simulink library "walkingRobotUtils"  (R2019a)
settings: Solver=VariableStepAuto  StartTime=0.0  StopTime=10.0  RelTol=1e-3
undefined symbols (not defined in the file): ankle_servo_kd, ankle_servo_ki, ankle_servo_kp, deriv_filter_coeff, joint_damping, joint_stiffness, lower_leg_length, max_torque, motion_time_constant, motor_constant, motor_inertia, upper_leg_length
libraries: nesl_utility x17, fl_lib x7, $bdroot x5, sm_lib x4, ee_lib x3, simulink x2, simulink_extras x2, robotcorelib x1, Multibody_Multiphysics_Lib x1
settings Model: Creator=scastro  LastModifiedBy=michaelmcgeehan
settings DataIOCC: ReturnWorkspaceOutputs=off
settings DebuggingCC: ArithmeticOperatorsInVariantConditions=warning
settings SFSimCC: SimUseLocalCustomCode=off
settings RTWCC: RTWUseLocalCustomCode=off
settings CodeAppCC: StateflowObjectComments=on

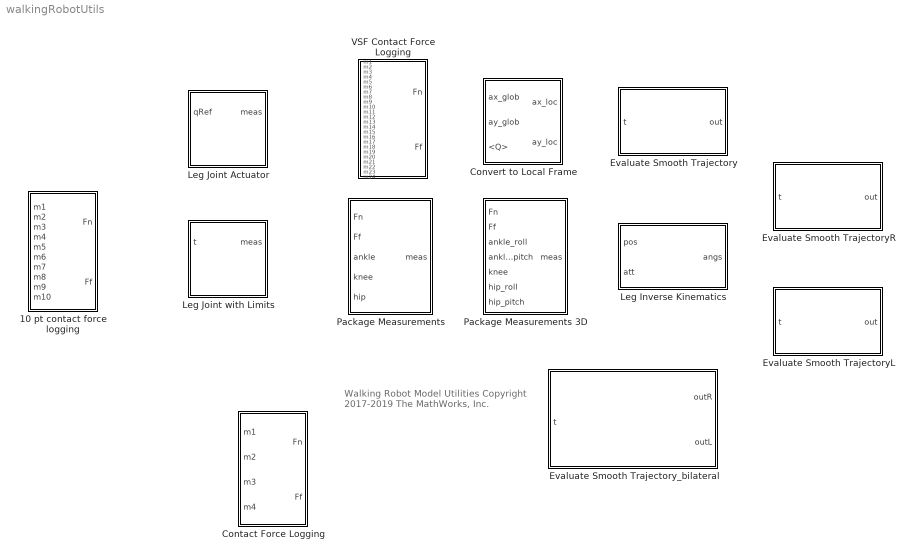
== system walkingRobotUtils ==
  note: Walking Robot Model Utilities
      |
      | Copyright 2017-2019 The MathWorks, Inc.
  10 pt contact force logging : Subsystem  AncestorBlock=walkingRobotUtils/VSF Contact Force Logging
  Contact Force Logging : Subsystem  AncestorBlock=walkingRobotUtils/VSF Contact Force Logging
  Convert to Local Frame : Subsystem
  Evaluate Smooth Trajectory : MATLAB Function  TreatAsAtomicUnit=on
  Evaluate Smooth TrajectoryL : MATLAB Function  TreatAsAtomicUnit=on
  Evaluate Smooth TrajectoryR : MATLAB Function  TreatAsAtomicUnit=on
  Evaluate Smooth Trajectory_bilateral : MATLAB Function  TreatAsAtomicUnit=on
  Leg Inverse Kinematics : MATLAB Function  TreatAsAtomicUnit=on
  Leg Joint Actuator : Subsystem  Variant=on  mask(Leg Joint Actuator){k=joint_stiffness, d=joint_damping, initAngle=0, Tf=motion_time_constant, Kp=ankle_servo_kp, Ki=ankle_servo_ki, Kd=ankle_servo_kd, N=deriv_filter_coeff, Tmax=max_torque}
      mask prompts: k "Joint Stiffness [N*m/rad]"; d "Joint Damping [N*m/(rad/s)]"; initAngle "Initial Joint Angle"; Tf "Motion Time Constant"; Kp "Servo Proportional Gain"; Ki "Servo Integral Gain"; Kd "Servo Derivative Gain"; N "Servo Filter Coefficient"; Tmax "Maximum Torque"
      mask DialogControl Container7 Prompt: Mechanics
      mask DialogControl Container4 Prompt: Controller
  Leg Joint with Limits : Subsystem  VariantControl=actuatorType == 2  mask(Leg Joint with Limits){k=1, d=0, initAngle=0, eqAngle=0, upperLimit=0, lowerLimit=-pi/8, jointLimitStiffness=100, jointLimitDamping=10}
      mask prompts: k "Joint Stiffness [N*m/rad]"; d "Joint Damping [N*m/(rad/s)]"; initAngle "Initial Angle [rad]"; eqAngle "Equilibrium Angle [rad]"; upperLimit "Upper Angle Limit [rad]"; lowerLimit "Lower Angle Limit [rad]"; jointLimitStiffness "Joint Limit Stiffness [N*m/rad]"; jointLimitDamping "Joint Limit Damping [N*m/(rad/s)]"
      mask help: Torque-actuated revolute joint with limits and instrumented measurements.
      mask DialogControl DynamicsTab Prompt: Dynamics
      mask DialogControl LimitsTab Prompt: Limits
  Package Measurements 3D : Subsystem
  Package Measurements : Subsystem
  VSF Contact Force Logging : Subsystem

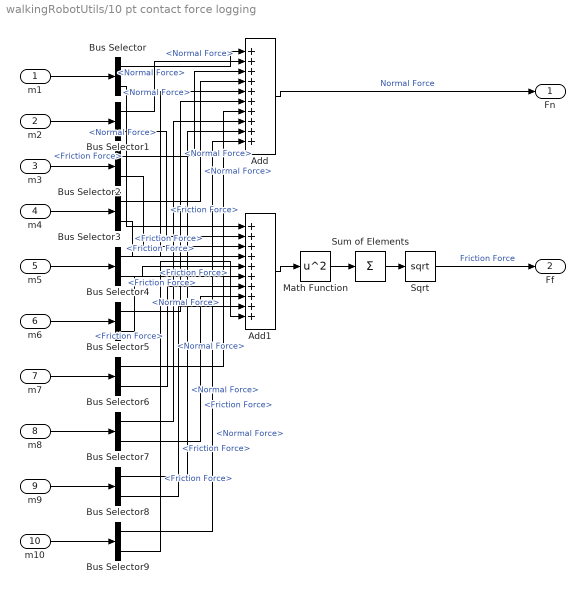
== system walkingRobotUtils/10 pt contact force logging ==
  m1 : Inport
  m2 : Inport  Port=2
  m3 : Inport  Port=3
  m4 : Inport  Port=4
  m5 : Inport  Port=5
  m6 : Inport  Port=6
  m7 : Inport  Port=7
  m8 : Inport  Port=8
  m9 : Inport  Port=9
  m10 : Inport  Port=10
  Add : Sum  Inputs=10
  Add1 : Sum  Inputs=10
  Bus Selector{,1..9} (10 alike) : BusSelector  OutputSignals=Normal Force,Friction Force
  Math Function : Math  Operator=square  SaturateOnIntegerOverflow=on
  Sqrt : Sqrt  SaturateOnIntegerOverflow=on
  Sum of Elements : Sum  Inputs=+
  Fn : Outport
  Ff : Outport  Port=2
  wires:
  m1/1 -> Bus Selector/1
  m2/1 -> Bus Selector1/1
  m3/1 -> Bus Selector2/1
  m4/1 -> Bus Selector3/1
  Bus Selector/1 -> Add/1  "<Normal Force>"
  Bus Selector1/1 -> Add/2  "<Normal Force>"
  Bus Selector2/1 -> Add/3  "<Normal Force>"
  Bus Selector3/1 -> Add/4  "<Normal Force>"
  Bus Selector/2 -> Add1/1  "<Friction Force>"
  Bus Selector1/2 -> Add1/2  "<Friction Force>"
  Bus Selector2/2 -> Add1/3  "<Friction Force>"
  Bus Selector3/2 -> Add1/4  "<Friction Force>"
  Add/1 -> Fn/1  "Normal Force"
  Add1/1 -> Math Function/1
  Math Function/1 -> Sum of Elements/1
  Sum of Elements/1 -> Sqrt/1
  Sqrt/1 -> Ff/1  "Friction Force"
  m5/1 -> Bus Selector4/1
  m6/1 -> Bus Selector5/1
  m7/1 -> Bus Selector6/1
  m8/1 -> Bus Selector7/1
  m9/1 -> Bus Selector8/1
  m10/1 -> Bus Selector9/1
  Bus Selector4/1 -> Add/5  "<Normal Force>"
  Bus Selector5/1 -> Add/6  "<Normal Force>"
  Bus Selector6/1 -> Add/7  "<Normal Force>"
  Bus Selector7/1 -> Add/8  "<Normal Force>"
  Bus Selector8/1 -> Add/9  "<Normal Force>"
  Bus Selector9/1 -> Add/10  "<Normal Force>"
  Bus Selector4/2 -> Add1/5  "<Friction Force>"
  Bus Selector5/2 -> Add1/6  "<Friction Force>"
  Bus Selector6/2 -> Add1/7  "<Friction Force>"
  Bus Selector7/2 -> Add1/8  "<Friction Force>"
  Bus Selector8/2 -> Add1/9  "<Friction Force>"
  Bus Selector9/2 -> Add1/10  "<Friction Force>"

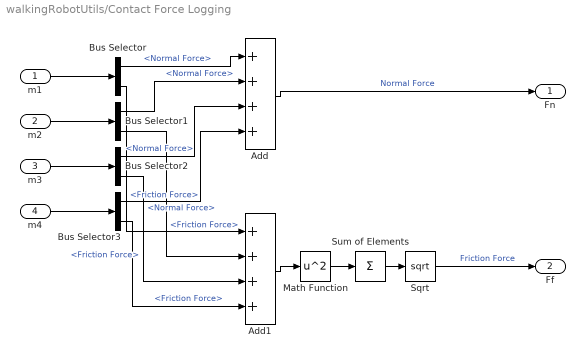
== system walkingRobotUtils/Contact Force Logging ==
  m1 : Inport
  m2 : Inport  Port=2
  m3 : Inport  Port=3
  m4 : Inport  Port=4
  Add : Sum  Inputs=4
  Add1 : Sum  Inputs=4
  Bus Selector{,1..3} (4 alike) : BusSelector  OutputSignals=Normal Force,Friction Force
  Math Function : Math  Operator=square  SaturateOnIntegerOverflow=on
  Sqrt : Sqrt  SaturateOnIntegerOverflow=on
  Sum of Elements : Sum  Inputs=+
  Fn : Outport
  Ff : Outport  Port=2
  wires:
  m1/1 -> Bus Selector/1
  m2/1 -> Bus Selector1/1
  m3/1 -> Bus Selector2/1
  m4/1 -> Bus Selector3/1
  Bus Selector/1 -> Add/1  "<Normal Force>"
  Bus Selector1/1 -> Add/2  "<Normal Force>"
  Bus Selector2/1 -> Add/3  "<Normal Force>"
  Bus Selector3/1 -> Add/4  "<Normal Force>"
  Bus Selector/2 -> Add1/1  "<Friction Force>"
  Bus Selector1/2 -> Add1/2  "<Friction Force>"
  Bus Selector2/2 -> Add1/3  "<Friction Force>"
  Bus Selector3/2 -> Add1/4  "<Friction Force>"
  Add/1 -> Fn/1  "Normal Force"
  Add1/1 -> Math Function/1
  Math Function/1 -> Sum of Elements/1
  Sum of Elements/1 -> Sqrt/1
  Sqrt/1 -> Ff/1  "Friction Force"

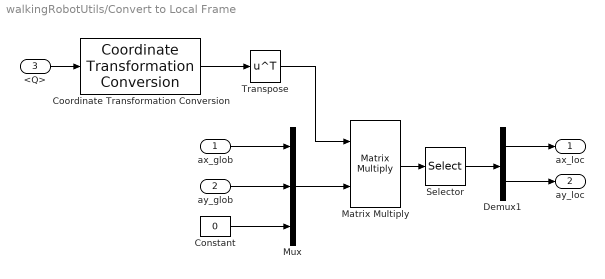
== system walkingRobotUtils/Convert to Local Frame ==
  ax_glob : Inport
  ay_glob : Inport  Port=2
  <Q> : Inport  Port=3
  Constant : Constant  Value=0
  Coordinate Transformation Conversion : robotcorelib/Coordinate Transformation Conversion  InputRepresentation=Quaternion  InputEulerSequence=ZYX  ShowTrVecInputPort=on  OutputRepresentation=Rotation Matrix  OutputEulerSequence=ZYX  ShowTrVecOutputPort=on  SimulateUsing=Interpreted execution
      settings: SourceProductBaseCode=RO
  Demux1 : Demux  Outputs=2
  Matrix Multiply : Product  Multiplication=Matrix(*)
  Mux : Mux  Inputs=3
  Selector : Selector  InputPortWidth=3  IndexOptions=Index vector (dialog)  Indices=[1 2]  OutputSizes=1
  Transpose : Math  Operator=transpose  SaturateOnIntegerOverflow=on
  ax_loc : Outport
  ay_loc : Outport  Port=2
  wires:
  Mux/1 -> Matrix Multiply/2
  Demux1/2 -> ay_loc/1
  ay_glob/1 -> Mux/2
  <Q>/1 -> Coordinate Transformation Conversion/1
  Selector/1 -> Demux1/1
  Matrix Multiply/1 -> Selector/1
  Constant/1 -> Mux/3
  ax_glob/1 -> Mux/1
  Demux1/1 -> ax_loc/1
  Coordinate Transformation Conversion/1 -> Transpose/1
  Transpose/1 -> Matrix Multiply/1

== system walkingRobotUtils/Leg Joint Actuator ==
  note: 1) Add Subsystem or Model blocks as valid variant choices.
      | 2) You cannot connect blocks at this level. At simulation, connectivity is automatically
      | determined, based on the active variant and port name matching.
  qRef : Inport
  Motion : Subsystem  VariantControl=actuatorType == 1
  Motor : Subsystem  VariantControl=actuatorType == 3
  Torque : Subsystem  VariantControl=actuatorType == 2
  B : PMIOPort  Side=Left
  F : PMIOPort  Port=2  Side=Right
  meas : Outport

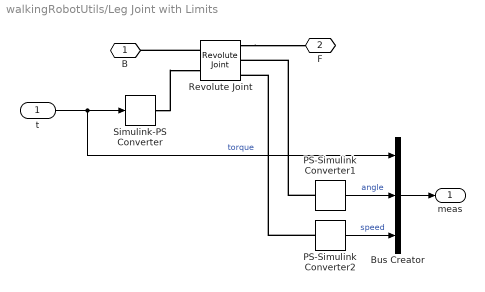
== system walkingRobotUtils/Leg Joint with Limits ==
  t : Inport
  Bus Creator : BusCreator  Inputs=3
  PS-Simulink Converter1 : nesl_utility/PS-Simulink Converter  PhysicalDomain=network_engine_domain  SubClassName=ps_output  LeftPortType=input  RightPortType=output  PseudoPeriodic=off  Frequencies=[]  Unit=rad  AffineConversion=off
  PS-Simulink Converter2 : nesl_utility/PS-Simulink Converter  PhysicalDomain=network_engine_domain  SubClassName=ps_output  LeftPortType=input  RightPortType=output  PseudoPeriodic=off  Frequencies=[]  Unit=rad/s  AffineConversion=off
  Revolute Joint : sm_lib/Joints/Revolute Joint  SenseConstraintForce=off  SenseConstraintForceX=off  SenseConstraintForceY=off  SenseConstraintForceZ=off  SenseConstraintTorque=off  SenseConstraintTorqueX=off  SenseConstraintTorqueY=off  SenseConstraintTorqueZ=off  SenseTotalForce=off  SenseTotalForceX=off  SenseTotalForceY=off  SenseTotalForceZ=off  SenseTotalTorque=off  SenseTotalTorqueX=off  SenseTotalTorqueY=off  SenseTotalTorqueZ=off  CompositeWrenchDir=FollowerOnBase  CompositeWrenchFrame=BaseFrame  EquilibriumPosition=eqAngle  EquilibriumPositionUnits=rad  SpringStiffness=k  SpringStiffnessUnits=N*m/rad  DampingCoefficient=d  DampingCoefficientUnits=N*m/(rad/s)  TorqueActuationMode=InputTorque  MotionActuationMode=ComputedMotion  SensePosition=on  SenseVelocity=on  SenseAcceleration=off  SenseTorqueForce=off  SenseLowerLimitTorqueForce=off  SenseUpperLimitTorqueForce=off  LowerLimitSpecify=on  LowerLimitBound=lowerLimit  LowerLimitBoundUnits=rad  LowerLimitStiffness=jointLimitStiffness  LowerLimitStiffnessUnits=N*m/rad  LowerLimitDamping=jointLimitDamping  LowerLimitDampingUnits=N*m/(rad/s)  LowerLimitTransitionRegionWidth=1  LowerLimitTransitionRegionWidthUnits=deg  UpperLimitSpecify=on  UpperLimitBound=upperLimit  UpperLimitBoundUnits=rad  UpperLimitStiffness=jointLimitStiffness  UpperLimitStiffnessUnits=N*m/rad  UpperLimitDamping=jointLimitDamping  UpperLimitDampingUnits=N*m/(rad/s)  UpperLimitTransitionRegionWidth=1  UpperLimitTransitionRegionWidthUnits=deg  PositionTargetSpecify=on  PositionTargetPriority=High  PositionTargetValue=initAngle  PositionTargetValueUnits=rad  VelocityTargetSpecify=off  VelocityTargetPriority=High  VelocityTargetValue=0  VelocityTargetValueUnits=deg/s
  Simulink-PS Converter : nesl_utility/Simulink-PS Converter  PhysicalDomain=network_engine_domain  SubClassName=ps_input  LeftPortType=input  RightPortType=output  PseudoPeriodic=off  Frequencies=[]  NoiseDistribution=none  NoiseParameters=[]  Unit=N*m  AffineConversion=off  FilteringAndDerivatives=provide  SimscapeFilterOrder=2  InputFilterTimeConstant=motion_time_constant  UdotUserProvided=0
  B : PMIOPort  Side=Left
  F : PMIOPort  Port=2  Side=Right
  meas : Outport
  wires:
  PS-Simulink Converter2/1 -> Bus Creator/3  "speed"
  t/1 -> Simulink-PS Converter/1, Bus Creator/1  "torque"
  Bus Creator/1 -> meas/1
  PS-Simulink Converter1/1 -> Bus Creator/2  "angle"
  connections:
  PS-Simulink Converter2/LConn1 -- Revolute Joint/RConn3
  Simulink-PS Converter/RConn1 -- Revolute Joint/LConn2
  Revolute Joint/RConn1 -- F/RConn1
  Revolute Joint/LConn1 -- B/RConn1
  PS-Simulink Converter1/LConn1 -- Revolute Joint/RConn2

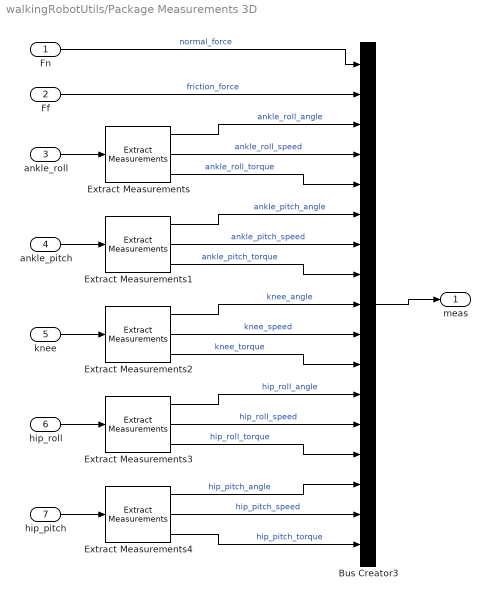
== system walkingRobotUtils/Package Measurements 3D ==
  Fn : Inport
  Ff : Inport  Port=2
  ankle_roll : Inport  Port=3
  ankle_pitch : Inport  Port=4
  knee : Inport  Port=5
  hip_roll : Inport  Port=6
  hip_pitch : Inport  Port=7
  Bus Creator3 : BusCreator  Inputs=17
  Extract Measurements{,1..4} (5 alike) : $bdroot/Package  Measurements/Extract Measurements  SystemSampleTime=-1
  meas : Outport
  wires:
  Extract Measurements4/2 -> Bus Creator3/16  "hip_pitch_speed"
  Extract Measurements3/2 -> Bus Creator3/13  "hip_roll_speed"
  Extract Measurements2/2 -> Bus Creator3/10  "knee_speed"
  Extract Measurements2/1 -> Bus Creator3/9  "knee_angle"
  Extract Measurements1/2 -> Bus Creator3/7  "ankle_pitch_speed"
  Extract Measurements/2 -> Bus Creator3/4  "ankle_roll_speed"
  Fn/1 -> Bus Creator3/1  "normal_force"
  Ff/1 -> Bus Creator3/2  "friction_force"
  Extract Measurements4/3 -> Bus Creator3/17  "hip_pitch_torque"
  Extract Measurements4/1 -> Bus Creator3/15  "hip_pitch_angle"
  Extract Measurements2/3 -> Bus Creator3/11  "knee_torque"
  hip_pitch/1 -> Extract Measurements4/1
  knee/1 -> Extract Measurements2/1
  Extract Measurements1/3 -> Bus Creator3/8  "ankle_pitch_torque"
  Extract Measurements1/1 -> Bus Creator3/6  "ankle_pitch_angle"
  ankle_pitch/1 -> Extract Measurements1/1
  Bus Creator3/1 -> meas/1
  ankle_roll/1 -> Extract Measurements/1
  Extract Measurements/1 -> Bus Creator3/3  "ankle_roll_angle"
  Extract Measurements/3 -> Bus Creator3/5  "ankle_roll_torque"
  hip_roll/1 -> Extract Measurements3/1
  Extract Measurements3/3 -> Bus Creator3/14  "hip_roll_torque"
  Extract Measurements3/1 -> Bus Creator3/12  "hip_roll_angle"

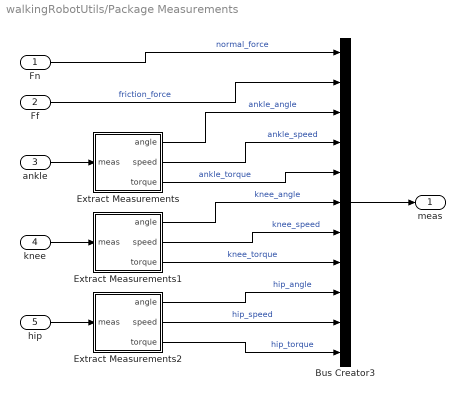
== system walkingRobotUtils/Package Measurements ==
  Fn : Inport
  Ff : Inport  Port=2
  ankle : Inport  Port=3
  knee : Inport  Port=4
  hip : Inport  Port=5
  Bus Creator3 : BusCreator  Inputs=11
  Extract Measurements : Subsystem
  Extract Measurements1 : Subsystem
  Extract Measurements2 : Subsystem
  meas : Outport
  wires:
  Extract Measurements2/2(speed) -> Bus Creator3/10  "hip_speed"
  Extract Measurements1/2(speed) -> Bus Creator3/7  "knee_speed"
  Extract Measurements/2(speed) -> Bus Creator3/4  "ankle_speed"
  Bus Creator3/1 -> meas/1
  ankle/1 -> Extract Measurements/1(meas)
  Extract Measurements/1(angle) -> Bus Creator3/3  "ankle_angle"
  Extract Measurements/3(torque) -> Bus Creator3/5  "ankle_torque"
  knee/1 -> Extract Measurements1/1(meas)
  hip/1 -> Extract Measurements2/1(meas)
  Extract Measurements1/1(angle) -> Bus Creator3/6  "knee_angle"
  Extract Measurements1/3(torque) -> Bus Creator3/8  "knee_torque"
  Extract Measurements2/1(angle) -> Bus Creator3/9  "hip_angle"
  Extract Measurements2/3(torque) -> Bus Creator3/11  "hip_torque"
  Ff/1 -> Bus Creator3/2  "friction_force"
  Fn/1 -> Bus Creator3/1  "normal_force"

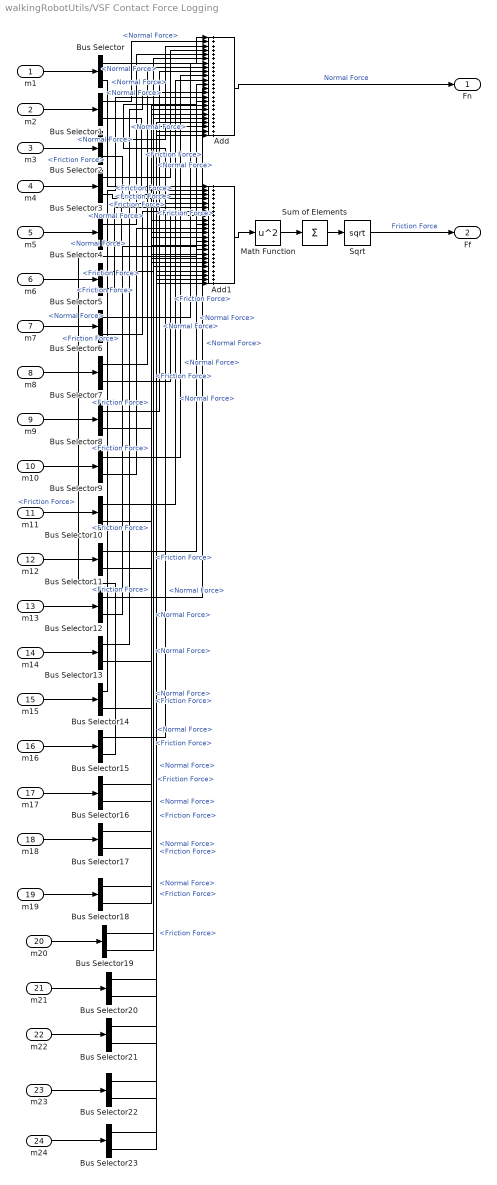
== system walkingRobotUtils/VSF Contact Force Logging ==
  m1 : Inport
  m2 : Inport  Port=2
  m3 : Inport  Port=3
  m4 : Inport  Port=4
  m5 : Inport  Port=5
  m6 : Inport  Port=6
  m7 : Inport  Port=7
  m8 : Inport  Port=8
  m9 : Inport  Port=9
  m10 : Inport  Port=10
  m11 : Inport  Port=11
  m12 : Inport  Port=12
  m13 : Inport  Port=13
  m14 : Inport  Port=14
  m15 : Inport  Port=15
  m16 : Inport  Port=16
  m17 : Inport  Port=17
  m18 : Inport  Port=18
  m19 : Inport  Port=19
  m20 : Inport  Port=20
  m21 : Inport  Port=21
  m22 : Inport  Port=22
  m23 : Inport  Port=23
  m24 : Inport  Port=24
  Add : Sum  Inputs=24
  Add1 : Sum  Inputs=24
  Bus Selector{,1..23} (24 alike) : BusSelector  OutputSignals=Normal Force,Friction Force
  Math Function : Math  Operator=square  SaturateOnIntegerOverflow=on
  Sqrt : Sqrt  SaturateOnIntegerOverflow=on
  Sum of Elements : Sum  Inputs=+
  Fn : Outport
  Ff : Outport  Port=2
  wires:
  m1/1 -> Bus Selector/1
  m2/1 -> Bus Selector1/1
  m3/1 -> Bus Selector2/1
  m4/1 -> Bus Selector3/1
  Bus Selector/1 -> Add/1  "<Normal Force>"
  Bus Selector1/1 -> Add/2  "<Normal Force>"
  Bus Selector2/1 -> Add/3  "<Normal Force>"
  Bus Selector3/1 -> Add/4  "<Normal Force>"
  Bus Selector/2 -> Add1/1  "<Friction Force>"
  Bus Selector1/2 -> Add1/2  "<Friction Force>"
  Bus Selector2/2 -> Add1/3  "<Friction Force>"
  Bus Selector3/2 -> Add1/4  "<Friction Force>"
  Add/1 -> Fn/1  "Normal Force"
  Add1/1 -> Math Function/1
  Math Function/1 -> Sum of Elements/1
  Sum of Elements/1 -> Sqrt/1
  Sqrt/1 -> Ff/1  "Friction Force"
  m5/1 -> Bus Selector4/1
  m6/1 -> Bus Selector5/1
  m7/1 -> Bus Selector6/1
  m8/1 -> Bus Selector7/1
  m9/1 -> Bus Selector8/1
  m10/1 -> Bus Selector9/1
  m11/1 -> Bus Selector10/1
  m12/1 -> Bus Selector11/1
  m13/1 -> Bus Selector12/1
  m14/1 -> Bus Selector13/1
  m15/1 -> Bus Selector14/1
  m16/1 -> Bus Selector15/1
  m17/1 -> Bus Selector16/1
  m18/1 -> Bus Selector17/1
  m19/1 -> Bus Selector18/1
  m20/1 -> Bus Selector19/1
  m21/1 -> Bus Selector20/1
  m22/1 -> Bus Selector21/1
  m23/1 -> Bus Selector22/1
  m24/1 -> Bus Selector23/1
  Bus Selector4/1 -> Add/5  "<Normal Force>"
  Bus Selector5/1 -> Add/6  "<Normal Force>"
  Bus Selector6/1 -> Add/7  "<Normal Force>"
  Bus Selector7/1 -> Add/8  "<Normal Force>"
  Bus Selector8/1 -> Add/9  "<Normal Force>"
  Bus Selector9/1 -> Add/10  "<Normal Force>"
  Bus Selector10/1 -> Add/11  "<Normal Force>"
  Bus Selector11/1 -> Add/12  "<Normal Force>"
  Bus Selector12/1 -> Add/13  "<Normal Force>"
  Bus Selector13/1 -> Add/14  "<Normal Force>"
  Bus Selector14/1 -> Add/15  "<Normal Force>"
  Bus Selector15/1 -> Add/16  "<Normal Force>"
  Bus Selector16/1 -> Add/17  "<Normal Force>"
  Bus Selector17/1 -> Add/18  "<Normal Force>"
  Bus Selector18/1 -> Add/19  "<Normal Force>"
  Bus Selector19/1 -> Add/20  "<Normal Force>"
  Bus Selector20/1 -> Add/21  "<Normal Force>"
  Bus Selector21/1 -> Add/22  "<Normal Force>"
  Bus Selector22/1 -> Add/23  "<Normal Force>"
  Bus Selector23/1 -> Add/24  "<Normal Force>"
  Bus Selector4/2 -> Add1/5  "<Friction Force>"
  Bus Selector5/2 -> Add1/6  "<Friction Force>"
  Bus Selector6/2 -> Add1/7  "<Friction Force>"
  Bus Selector7/2 -> Add1/8  "<Friction Force>"
  Bus Selector8/2 -> Add1/9  "<Friction Force>"
  Bus Selector9/2 -> Add1/10  "<Friction Force>"
  Bus Selector10/2 -> Add1/11  "<Friction Force>"
  Bus Selector14/2 -> Add1/12  "<Friction Force>"
  Bus Selector11/2 -> Add1/13  "<Friction Force>"
  Bus Selector12/2 -> Add1/14  "<Friction Force>"
  Bus Selector13/2 -> Add1/15  "<Friction Force>"
  Bus Selector15/2 -> Add1/16  "<Friction Force>"
  Bus Selector16/2 -> Add1/17  "<Friction Force>"
  Bus Selector17/2 -> Add1/18  "<Friction Force>"
  Bus Selector18/2 -> Add1/19  "<Friction Force>"
  Bus Selector19/2 -> Add1/20  "<Friction Force>"
  Bus Selector20/2 -> Add1/21  "<Friction Force>"
  Bus Selector21/2 -> Add1/22  "<Friction Force>"
  Bus Selector22/2 -> Add1/23  "<Friction Force>"
  Bus Selector23/2 -> Add1/24  "<Friction Force>"

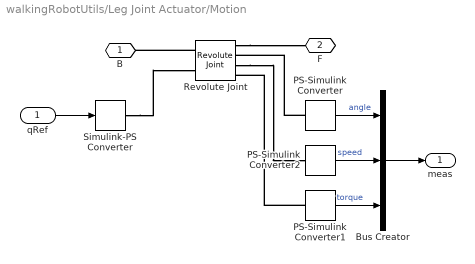
== system walkingRobotUtils/Leg Joint Actuator/Motion ==
  qRef : Inport
  Bus Creator : BusCreator  Inputs=3
  PS-Simulink Converter : nesl_utility/PS-Simulink Converter  PhysicalDomain=network_engine_domain  SubClassName=ps_output  LeftPortType=input  RightPortType=output  PseudoPeriodic=off  Frequencies=[]  Unit=rad  AffineConversion=off
  PS-Simulink Converter1 : nesl_utility/PS-Simulink Converter  PhysicalDomain=network_engine_domain  SubClassName=ps_output  LeftPortType=input  RightPortType=output  PseudoPeriodic=off  Frequencies=[]  Unit=N*m  AffineConversion=off
  PS-Simulink Converter2 : nesl_utility/PS-Simulink Converter  PhysicalDomain=network_engine_domain  SubClassName=ps_output  LeftPortType=input  RightPortType=output  PseudoPeriodic=off  Frequencies=[]  Unit=rad/s  AffineConversion=off
  Revolute Joint : sm_lib/Joints/Revolute Joint  SenseConstraintForce=off  SenseConstraintForceX=off  SenseConstraintForceY=off  SenseConstraintForceZ=off  SenseConstraintTorque=off  SenseConstraintTorqueX=off  SenseConstraintTorqueY=off  SenseConstraintTorqueZ=off  SenseTotalForce=off  SenseTotalForceX=off  SenseTotalForceY=off  SenseTotalForceZ=off  SenseTotalTorque=off  SenseTotalTorqueX=off  SenseTotalTorqueY=off  SenseTotalTorqueZ=off  CompositeWrenchDir=FollowerOnBase  CompositeWrenchFrame=BaseFrame  EquilibriumPosition=0  EquilibriumPositionUnits=deg  SpringStiffness=k  SpringStiffnessUnits=N*m/rad  DampingCoefficient=d  DampingCoefficientUnits=N*m/(rad/s)  TorqueActuationMode=ComputedTorque  MotionActuationMode=InputMotion  SensePosition=on  SenseVelocity=on  SenseAcceleration=off  SenseTorqueForce=on  SenseLowerLimitTorqueForce=off  SenseUpperLimitTorqueForce=off  LowerLimitSpecify=off  LowerLimitBound=-90  LowerLimitBoundUnits=deg  LowerLimitStiffness=1e4  LowerLimitStiffnessUnits=N*m/deg  LowerLimitDamping=10  LowerLimitDampingUnits=N*m/(deg/s)  LowerLimitTransitionRegionWidth=0.1  LowerLimitTransitionRegionWidthUnits=deg  UpperLimitSpecify=off  UpperLimitBound=90  UpperLimitBoundUnits=deg  UpperLimitStiffness=1e4  UpperLimitStiffnessUnits=N*m/deg  UpperLimitDamping=10  UpperLimitDampingUnits=N*m/(deg/s)  UpperLimitTransitionRegionWidth=0.1  UpperLimitTransitionRegionWidthUnits=deg  PositionTargetSpecify=off  PositionTargetPriority=High  PositionTargetValue=0  PositionTargetValueUnits=rad  VelocityTargetSpecify=off  VelocityTargetPriority=High  VelocityTargetValue=0  VelocityTargetValueUnits=deg/s
  Simulink-PS Converter : nesl_utility/Simulink-PS Converter  PhysicalDomain=network_engine_domain  SubClassName=ps_input  LeftPortType=input  RightPortType=output  PseudoPeriodic=off  Frequencies=[]  NoiseDistribution=none  NoiseParameters=[]  Unit=rad  AffineConversion=off  FilteringAndDerivatives=filter  SimscapeFilterOrder=2  InputFilterTimeConstant=Tf  UdotUserProvided=0
  B : PMIOPort  Side=Left
  F : PMIOPort  Port=2  Side=Right
  meas : Outport
  wires:
  qRef/1 -> Simulink-PS Converter/1
  PS-Simulink Converter/1 -> Bus Creator/1  "angle"
  PS-Simulink Converter1/1 -> Bus Creator/3  "torque"
  Bus Creator/1 -> meas/1
  PS-Simulink Converter2/1 -> Bus Creator/2  "speed"
  connections:
  Revolute Joint/RConn1 -- F/RConn1
  Revolute Joint/LConn1 -- B/RConn1
  Simulink-PS Converter/RConn1 -- Revolute Joint/LConn2
  PS-Simulink Converter/LConn1 -- Revolute Joint/RConn2
  PS-Simulink Converter1/LConn1 -- Revolute Joint/RConn4
  Revolute Joint/RConn3 -- PS-Simulink Converter2/LConn1

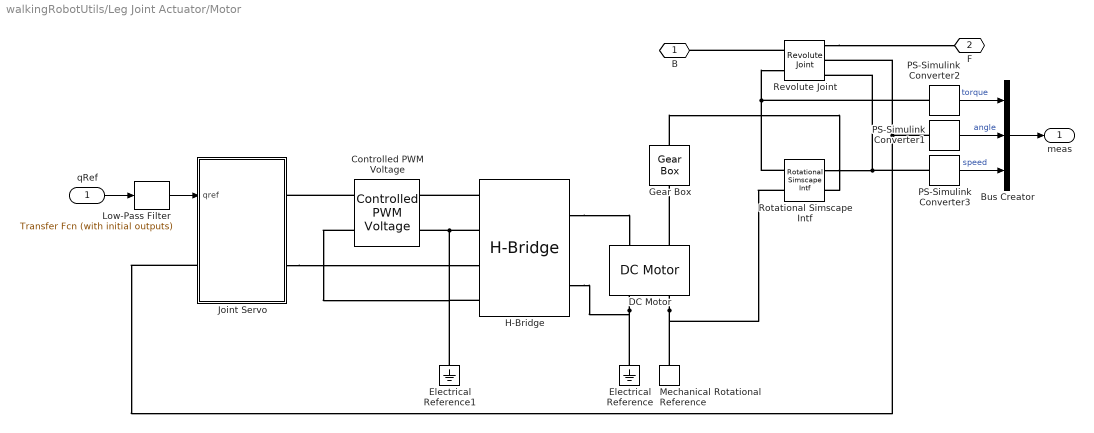
== system walkingRobotUtils/Leg Joint Actuator/Motor ==
  qRef : Inport
  Bus Creator : BusCreator  Inputs=3
  Controlled PWM Voltage : ee_lib/Integrated Circuits/Controlled PWM Voltage  F=1000 Hz  TD=0 s  pulse_width_offset=0 s  pulse_min=0 s  Vmin=0 V  Vmax=20 V  Vm=5 V  pwm_or_av=2  event_type=1  sample_time=1e-6 s  u_min=0  u_max=1
      settings: SourceProductName=Simscape Electrical
  DC Motor : ee_lib/Electromechanical/Brushed Motors/DC Motor  parameterization=1  Ra=motor_resistance Ohm  La=motor_inductance H  emf_or_torque=2  Kv=0.01 V/rpm  Ki=motor_constant N*m/A  T_stall=2.4e-4 N*m  w_max=1.91e+4 rpm  w_rated=1.5e+4 rpm  P_rated=0.08 W  V_rated=1.5 V  J=motor_inertia kg*m^2  lam_param=1  lam=motor_damping N*m/(rad/s)  i_noload=0 A  V_i_noload=1.5 V  speed0=0 rpm  alpha=3.93e-3 1/K  Tmeas=25 degC  thermal_mass=100 J/K  initial_temperature=25 degC
      settings: SourceProductName=Simscape Electrical
  Electrical Reference : fl_lib/Electrical/Electrical Elements/Electrical Reference
  Electrical Reference1 : fl_lib/Electrical/Electrical Elements/Electrical Reference
  Gear Box : fl_lib/Mechanical/Mechanisms/Gear Box  ratio=gear_ratio  t_in_specify=off  t_in_priority=None  t_in=0 N*m  t_in_nominal_specify=off  t_in_nominal_unit=N*m  t_in_nominal_value=1  t_out_specify=off  t_out_priority=None  t_out=0 N*m  t_out_nominal_specify=off  t_out_nominal_unit=N*m  t_out_nominal_value=1
  H-Bridge : ee_lib/Semiconductors & Converters/Converters/H-Bridge  Venable=1e-3 V  Vmax=5 V  Vreverse=2.5 V  Vbrake=2.5 V  Vm=24 V  pwm_or_av=2  discontinuous=0  freewheeling_mode=1  freewheeling_mode_disc=1  Ron=1e-3 Ohm  Don=1e-3 Ohm  Rload=10 Ohm  Lload=1e-5 H  F=10 kHz  thermal_mass=100 J/K  initial_temperature=298.15 K  Ron2=0.1 Ohm  Don2=0.05 Ohm  Tmeas=298.15 K  Tmeas2=398.15 K
      settings: SourceProductName=Simscape Electrical
  Joint Servo : Subsystem
  Low-Pass Filter : simulink_extras/Additional Linear/Transfer Fcn (with initial outputs)  N=[(1/motion_time_constant)^2]  D=[1 2/motion_time_constant (1/motion_time_constant)^2]  Y0=initAngle  U0=initAngle
  Mechanical Rotational Reference : fl_lib/Mechanical/Rotational Elements/Mechanical Rotational Reference
  PS-Simulink Converter1 : nesl_utility/PS-Simulink Converter  PhysicalDomain=network_engine_domain  SubClassName=ps_output  LeftPortType=input  RightPortType=output  PseudoPeriodic=off  Frequencies=[]  Unit=deg  AffineConversion=off
  PS-Simulink Converter2 : nesl_utility/PS-Simulink Converter  PhysicalDomain=network_engine_domain  SubClassName=ps_output  LeftPortType=input  RightPortType=output  PseudoPeriodic=off  Frequencies=[]  Unit=N*m  AffineConversion=off
  PS-Simulink Converter3 : nesl_utility/PS-Simulink Converter  PhysicalDomain=network_engine_domain  SubClassName=ps_output  LeftPortType=input  RightPortType=output  PseudoPeriodic=off  Frequencies=[]  Unit=rad/s  AffineConversion=off
  Revolute Joint : sm_lib/Joints/Revolute Joint  SenseConstraintForce=off  SenseConstraintForceX=off  SenseConstraintForceY=off  SenseConstraintForceZ=off  SenseConstraintTorque=off  SenseConstraintTorqueX=off  SenseConstraintTorqueY=off  SenseConstraintTorqueZ=off  SenseTotalForce=off  SenseTotalForceX=off  SenseTotalForceY=off  SenseTotalForceZ=off  SenseTotalTorque=off  SenseTotalTorqueX=off  SenseTotalTorqueY=off  SenseTotalTorqueZ=off  CompositeWrenchDir=FollowerOnBase  CompositeWrenchFrame=BaseFrame  EquilibriumPosition=0  EquilibriumPositionUnits=deg  SpringStiffness=k  SpringStiffnessUnits=N*m/rad  DampingCoefficient=d  DampingCoefficientUnits=N*m/(rad/s)  TorqueActuationMode=InputTorque  MotionActuationMode=ComputedMotion  SensePosition=on  SenseVelocity=on  SenseAcceleration=off  SenseTorqueForce=off  SenseLowerLimitTorqueForce=off  SenseUpperLimitTorqueForce=off  LowerLimitSpecify=off  LowerLimitBound=-90  LowerLimitBoundUnits=deg  LowerLimitStiffness=1e4  LowerLimitStiffnessUnits=N*m/deg  LowerLimitDamping=10  LowerLimitDampingUnits=N*m/(deg/s)  LowerLimitTransitionRegionWidth=0.1  LowerLimitTransitionRegionWidthUnits=deg  UpperLimitSpecify=off  UpperLimitBound=90  UpperLimitBoundUnits=deg  UpperLimitStiffness=1e4  UpperLimitStiffnessUnits=N*m/deg  UpperLimitDamping=10  UpperLimitDampingUnits=N*m/(deg/s)  UpperLimitTransitionRegionWidth=0.1  UpperLimitTransitionRegionWidthUnits=deg  PositionTargetSpecify=on  PositionTargetPriority=High  PositionTargetValue=initAngle  PositionTargetValueUnits=rad  VelocityTargetSpecify=off  VelocityTargetPriority=High  VelocityTargetValue=0  VelocityTargetValueUnits=deg/s
  Rotational Simscape Intf : Multibody_Multiphysics_Lib/Interfaces/Rotational Simscape Intf  SystemSampleTime=-1
      settings: SourceProductName=Simscape Multibody Multiphysics Library
  B : PMIOPort  Side=Left
  F : PMIOPort  Port=2  Side=Right
  meas : Outport
  wires:
  Low-Pass Filter/1 -> Joint Servo/1(qref)
  qRef/1 -> Low-Pass Filter/1
  PS-Simulink Converter2/1 -> Bus Creator/1  "torque"
  Bus Creator/1 -> meas/1
  PS-Simulink Converter1/1 -> Bus Creator/2  "angle"
  PS-Simulink Converter3/1 -> Bus Creator/3  "speed"
  connections:
  DC Motor/LConn2 -- Gear Box/LConn1
  H-Bridge/RConn1 -- DC Motor/LConn1
  Joint Servo/RConn2 -- H-Bridge/LConn3
  Rotational Simscape Intf/RConn1 -- Revolute Joint/RConn3 -- PS-Simulink Converter3/LConn1
  DC Motor/RConn1 -- H-Bridge/RConn2 -- Electrical Reference/LConn1
  Controlled PWM Voltage/LConn1 -- Joint Servo/RConn1
  H-Bridge/LConn1 -- Controlled PWM Voltage/RConn1
  H-Bridge/LConn2 -- Controlled PWM Voltage/RConn2 -- Controlled PWM Voltage/LConn2 -- H-Bridge/LConn4 -- Electrical Reference1/LConn1
  Gear Box/RConn1 -- Rotational Simscape Intf/RConn2
  DC Motor/RConn2 -- Rotational Simscape Intf/LConn2 -- Mechanical Rotational Reference/LConn1
  Joint Servo/LConn1 -- Revolute Joint/RConn2 -- PS-Simulink Converter1/LConn1
  Revolute Joint/LConn1 -- B/RConn1
  Revolute Joint/RConn1 -- F/RConn1
  Rotational Simscape Intf/LConn1 -- Revolute Joint/LConn2 -- PS-Simulink Converter2/LConn1

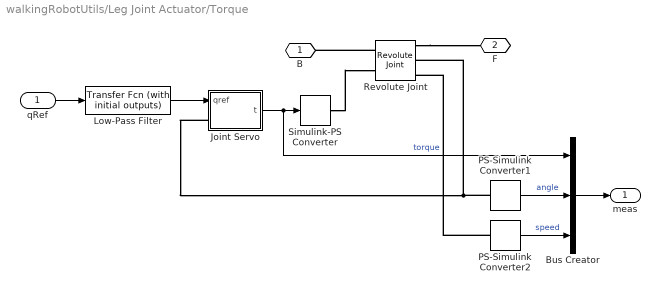
== system walkingRobotUtils/Leg Joint Actuator/Torque ==
  qRef : Inport
  Bus Creator : BusCreator  Inputs=3
  Joint Servo : Subsystem
  Low-Pass Filter : simulink_extras/Additional Linear/Transfer Fcn (with initial outputs)  N=[(1/motion_time_constant)^2]  D=[1 2/motion_time_constant (1/motion_time_constant)^2]  Y0=initAngle  U0=initAngle
  PS-Simulink Converter1 : nesl_utility/PS-Simulink Converter  PhysicalDomain=network_engine_domain  SubClassName=ps_output  LeftPortType=input  RightPortType=output  PseudoPeriodic=off  Frequencies=[]  Unit=deg  AffineConversion=off
  PS-Simulink Converter2 : nesl_utility/PS-Simulink Converter  PhysicalDomain=network_engine_domain  SubClassName=ps_output  LeftPortType=input  RightPortType=output  PseudoPeriodic=off  Frequencies=[]  Unit=rad/s  AffineConversion=off
  Revolute Joint : sm_lib/Joints/Revolute Joint  SenseConstraintForce=off  SenseConstraintForceX=off  SenseConstraintForceY=off  SenseConstraintForceZ=off  SenseConstraintTorque=off  SenseConstraintTorqueX=off  SenseConstraintTorqueY=off  SenseConstraintTorqueZ=off  SenseTotalForce=off  SenseTotalForceX=off  SenseTotalForceY=off  SenseTotalForceZ=off  SenseTotalTorque=off  SenseTotalTorqueX=off  SenseTotalTorqueY=off  SenseTotalTorqueZ=off  CompositeWrenchDir=FollowerOnBase  CompositeWrenchFrame=BaseFrame  EquilibriumPosition=0  EquilibriumPositionUnits=deg  SpringStiffness=k  SpringStiffnessUnits=N*m/rad  DampingCoefficient=d  DampingCoefficientUnits=N*m/(rad/s)  TorqueActuationMode=InputTorque  MotionActuationMode=ComputedMotion  SensePosition=on  SenseVelocity=on  SenseAcceleration=off  SenseTorqueForce=off  SenseLowerLimitTorqueForce=off  SenseUpperLimitTorqueForce=off  LowerLimitSpecify=off  LowerLimitBound=-90  LowerLimitBoundUnits=deg  LowerLimitStiffness=1e4  LowerLimitStiffnessUnits=N*m/deg  LowerLimitDamping=10  LowerLimitDampingUnits=N*m/(deg/s)  LowerLimitTransitionRegionWidth=0.1  LowerLimitTransitionRegionWidthUnits=deg  UpperLimitSpecify=off  UpperLimitBound=90  UpperLimitBoundUnits=deg  UpperLimitStiffness=1e4  UpperLimitStiffnessUnits=N*m/deg  UpperLimitDamping=10  UpperLimitDampingUnits=N*m/(deg/s)  UpperLimitTransitionRegionWidth=0.1  UpperLimitTransitionRegionWidthUnits=deg  PositionTargetSpecify=on  PositionTargetPriority=High  PositionTargetValue=initAngle  PositionTargetValueUnits=rad  VelocityTargetSpecify=off  VelocityTargetPriority=High  VelocityTargetValue=0  VelocityTargetValueUnits=deg/s
  Simulink-PS Converter : nesl_utility/Simulink-PS Converter  PhysicalDomain=network_engine_domain  SubClassName=ps_input  LeftPortType=input  RightPortType=output  PseudoPeriodic=off  Frequencies=[]  NoiseDistribution=none  NoiseParameters=[]  Unit=N*m  AffineConversion=off  FilteringAndDerivatives=provide  SimscapeFilterOrder=2  InputFilterTimeConstant=motion_time_constant  UdotUserProvided=0
  B : PMIOPort  Side=Left
  F : PMIOPort  Port=2  Side=Right
  meas : Outport
  wires:
  qRef/1 -> Low-Pass Filter/1
  Low-Pass Filter/1 -> Joint Servo/1(qref)
  PS-Simulink Converter1/1 -> Bus Creator/2  "angle"
  Bus Creator/1 -> meas/1
  Joint Servo/1(t) -> Bus Creator/1, Simulink-PS Converter/1  "torque"
  PS-Simulink Converter2/1 -> Bus Creator/3  "speed"
  connections:
  Joint Servo/LConn1 -- Revolute Joint/RConn2 -- PS-Simulink Converter1/LConn1
  Revolute Joint/LConn1 -- B/RConn1
  Revolute Joint/RConn1 -- F/RConn1
  Simulink-PS Converter/RConn1 -- Revolute Joint/LConn2
  PS-Simulink Converter2/LConn1 -- Revolute Joint/RConn3

== system walkingRobotUtils/Package Measurements/Extract Measurements ==
  meas : Inport
  Bus Selector : BusSelector  OutputSignals=angle,speed,torque
  angle : Outport
  speed : Outport  Port=2
  torque : Outport  Port=3
  wires:
  Bus Selector/2 -> speed/1  "<speed>"
  Bus Selector/3 -> torque/1  "<torque>"
  meas/1 -> Bus Selector/1
  Bus Selector/1 -> angle/1  "<angle>"

== system walkingRobotUtils/Package Measurements/Extract Measurements1 ==
  meas : Inport
  Bus Selector : BusSelector  OutputSignals=angle,speed,torque
  angle : Outport
  speed : Outport  Port=2
  torque : Outport  Port=3
  wires:
  Bus Selector/1 -> angle/1  "<angle>"
  meas/1 -> Bus Selector/1
  Bus Selector/3 -> torque/1  "<torque>"
  Bus Selector/2 -> speed/1  "<speed>"

== system walkingRobotUtils/Package Measurements/Extract Measurements2 ==
  meas : Inport
  Bus Selector : BusSelector  OutputSignals=angle,speed,torque
  angle : Outport
  speed : Outport  Port=2
  torque : Outport  Port=3
  wires:
  Bus Selector/2 -> speed/1  "<speed>"
  Bus Selector/3 -> torque/1  "<torque>"
  meas/1 -> Bus Selector/1
  Bus Selector/1 -> angle/1  "<angle>"

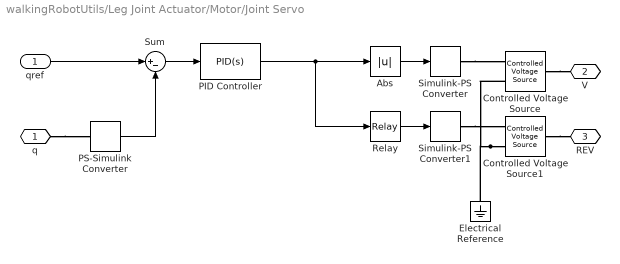
== system walkingRobotUtils/Leg Joint Actuator/Motor/Joint Servo ==
  qref : Inport
  Abs : Abs  ZeroCross=off
  Controlled Voltage Source : fl_lib/Electrical/Electrical Sources/Controlled Voltage Source
  Controlled Voltage Source1 : fl_lib/Electrical/Electrical Sources/Controlled Voltage Source
  Electrical Reference : fl_lib/Electrical/Electrical Elements/Electrical Reference
  PID Controller : simulink/Continuous/PID Controller  Controller=PID  Form=Parallel  TimeDomain=Continuous-time  SampleTime=-1  IntegratorMethod=Forward Euler  FilterMethod=Forward Euler  ControllerParametersSource=internal  P=Kp  I=Ki  D=Kd  UseFilter=on  N=N  ZeroCross=off  InitialConditionSource=internal  InitialConditionForIntegrator=0  InitialConditionForFilter=0  DifferentiatorICPrevScaledInput=0  ExternalReset=none  TrackingMode=off  Kt=1  LimitOutput=on  UpperSaturationLimit=Tmax  LowerSaturationLimit=-Tmax  LinearizeAsGain=on  AntiWindupMode=clamping  Kb=1  POutMin=[]  POutMax=[]  IOutMin=[]  IOutMax=[]  DOutMin=[]  DOutMax=[]  NOutMin=[]  NOutMax=[]  SumOutMin=[]  SumOutMax=[]  SaturationOutMin=[]  SaturationOutMax=[]  PParamMin=[]  PParamMax=[]  IParamMin=[]  IParamMax=[]  DParamMin=[]  DParamMax=[]  NParamMin=[]  NParamMax=[]  KbParamMin=[]  KbParamMax=[]  KtParamMin=[]  KtParamMax=[]  KbOutMin=[]  KbOutMax=[]  KtOutMin=[]  KtOutMax=[]  IntegratorOutMin=[]  IntegratorOutMax=[]  FilterOutMin=[]  FilterOutMax=[]  SumI1OutMin=[]  SumI1OutMax=[]  SumI2OutMin=[]  SumI2OutMax=[]  SumI3OutMin=[]  SumI3OutMax=[]  SumDOutMin=[]  SumDOutMax=[]  DifferentiatorOutMin=[]  DifferentiatorOutMax=[]  IntegratorContinuousStateAttributes=''  IntegratorStateMustResolveToSignalObject=off  IntegratorRTWStateStorageClass=Auto  FilterContinuousStateAttributes=''  FilterStateMustResolveToSignalObject=off  FilterRTWStateStorageClass=Auto
  PS-Simulink Converter : nesl_utility/PS-Simulink Converter  PhysicalDomain=network_engine_domain  SubClassName=ps_output  LeftPortType=input  RightPortType=output  PseudoPeriodic=off  Frequencies=[]  Unit=rad  AffineConversion=off
  Relay : Relay  OnSwitchValue=1e-3  OffSwitchValue=-1e-3  OnOutputValue=0  OffOutputValue=5  ZeroCross=off
  Simulink-PS Converter : nesl_utility/Simulink-PS Converter  PhysicalDomain=network_engine_domain  SubClassName=ps_input  LeftPortType=input  RightPortType=output  PseudoPeriodic=off  Frequencies=[]  NoiseDistribution=none  NoiseParameters=[]  Unit=1  AffineConversion=off  FilteringAndDerivatives=provide  SimscapeFilterOrder=1  InputFilterTimeConstant=0.005  UdotUserProvided=0
  Simulink-PS Converter1 : nesl_utility/Simulink-PS Converter  PhysicalDomain=network_engine_domain  SubClassName=ps_input  LeftPortType=input  RightPortType=output  PseudoPeriodic=off  Frequencies=[]  NoiseDistribution=none  NoiseParameters=[]  Unit=1  AffineConversion=off  FilteringAndDerivatives=provide  SimscapeFilterOrder=1  InputFilterTimeConstant=0.005  UdotUserProvided=0
  Sum : Sum  Inputs=|+-
  q : PMIOPort  Side=Left
  V : PMIOPort  Port=2  Side=Right
  REV : PMIOPort  Port=3  Side=Right
  wires:
  Relay/1 -> Simulink-PS Converter1/1
  Abs/1 -> Simulink-PS Converter/1
  Sum/1 -> PID Controller/1
  PS-Simulink Converter/1 -> Sum/2
  qref/1 -> Sum/1
  PID Controller/1 -> Relay/1, Abs/1
  connections:
  Simulink-PS Converter1/RConn1 -- Controlled Voltage Source1/RConn1
  Controlled Voltage Source1/LConn1 -- REV/RConn1
  Controlled Voltage Source1/RConn2 -- Controlled Voltage Source/RConn2 -- Electrical Reference/LConn1
  Controlled Voltage Source/LConn1 -- V/RConn1
  Simulink-PS Converter/RConn1 -- Controlled Voltage Source/RConn1
  q/RConn1 -- PS-Simulink Converter/LConn1

== system walkingRobotUtils/Leg Joint Actuator/Torque/Joint Servo ==
  qref : Inport
  PID Controller : simulink/Continuous/PID Controller  Controller=PID  Form=Parallel  TimeDomain=Continuous-time  SampleTime=-1  IntegratorMethod=Forward Euler  FilterMethod=Forward Euler  ControllerParametersSource=internal  P=Kp  I=Ki  D=Kd  UseFilter=on  N=N  ZeroCross=off  InitialConditionSource=internal  InitialConditionForIntegrator=0  InitialConditionForFilter=0  DifferentiatorICPrevScaledInput=0  ExternalReset=none  TrackingMode=off  Kt=1  LimitOutput=on  UpperSaturationLimit=Tmax  LowerSaturationLimit=-Tmax  LinearizeAsGain=on  AntiWindupMode=clamping  Kb=1  POutMin=[]  POutMax=[]  IOutMin=[]  IOutMax=[]  DOutMin=[]  DOutMax=[]  NOutMin=[]  NOutMax=[]  SumOutMin=[]  SumOutMax=[]  SaturationOutMin=[]  SaturationOutMax=[]  PParamMin=[]  PParamMax=[]  IParamMin=[]  IParamMax=[]  DParamMin=[]  DParamMax=[]  NParamMin=[]  NParamMax=[]  KbParamMin=[]  KbParamMax=[]  KtParamMin=[]  KtParamMax=[]  KbOutMin=[]  KbOutMax=[]  KtOutMin=[]  KtOutMax=[]  IntegratorOutMin=[]  IntegratorOutMax=[]  FilterOutMin=[]  FilterOutMax=[]  SumI1OutMin=[]  SumI1OutMax=[]  SumI2OutMin=[]  SumI2OutMax=[]  SumI3OutMin=[]  SumI3OutMax=[]  SumDOutMin=[]  SumDOutMax=[]  DifferentiatorOutMin=[]  DifferentiatorOutMax=[]  IntegratorContinuousStateAttributes=''  IntegratorStateMustResolveToSignalObject=off  IntegratorRTWStateStorageClass=Auto  FilterContinuousStateAttributes=''  FilterStateMustResolveToSignalObject=off  FilterRTWStateStorageClass=Auto
  PS-Simulink Converter : nesl_utility/PS-Simulink Converter  PhysicalDomain=network_engine_domain  SubClassName=ps_output  LeftPortType=input  RightPortType=output  PseudoPeriodic=off  Frequencies=[]  Unit=rad  AffineConversion=off
  Sum : Sum  Inputs=|+-
  q : PMIOPort  Side=Left
  t : Outport
  wires:
  qref/1 -> Sum/1
  PS-Simulink Converter/1 -> Sum/2
  Sum/1 -> PID Controller/1
  PID Controller/1 -> t/1
  connections:
  q/RConn1 -- PS-Simulink Converter/LConn1

== matlab function walkingRobotUtils/Evaluate Smooth Trajectory_bilateral ==
  data: t input; outR output; curveData parameter; outL output
function [outR,outL] = smoothTraj(t,curveData)

    % Call evalSmoothTrajectory function
    outR = evalSmoothTrajectory(curveData.R,t);
    outL = evalSmoothTrajectory(curveData.L,t);

end

== matlab function walkingRobotUtils/Leg Inverse Kinematics ==
  settings: updateMethod=DISCRETE
  data: pos input; angs output; att input; upper_leg_length parameter; lower_leg_length parameter
function angs = invKin3D(pos, att, upper_leg_length, lower_leg_length)

    % Unpack
    yaw = att(1);
    pitch = att(2);
    roll = att(3);
    x = pos(1);
    y = pos(2);
    z = pos(3);
    
    % Compute the hip angle
    hipRoll = -atan2(y,-z);
    
    % Call symbolic generated function for 2D leg
    zMod = z/cos(hipRoll);
    
    maxMag = 0.1975;
    mag = sqrt(x^2 + zMod^2);
    if sqrt(x^2 + zMod^2) > maxMag
        x = x*maxMag/mag;
        zMod = zMod*maxMag/mag;
    end
    
    theta = legInvKin(upper_leg_length/100,lower_leg_length/100,-x,zMod);
    
    % Address multiple outputs
    if size(theta,1) == 2
       if theta(1,2) < 0
          hipPitch = theta(2,1);
          kneePitch = theta(2,2);
       else
          hipPitch = theta(1,1);
          kneePitch = theta(1,2);
       end
    else
        hipPitch = theta(1);
        kneePitch = theta(2);
    end
    
    % Compensate for torso attitude and set ankle angles
    hipPitch = hipPitch + pitch;
    anklePitch = -kneePitch - hipPitch;
    ankleRoll  = roll - hipRoll;
    
    % Pack
    angs = [ankleRoll; anklePitch; kneePitch; hipRoll; hipPitch];
    
end

== matlab function walkingRobotUtils/Evaluate Smooth TrajectoryR ==
  data: t input; out output; curveDataR parameter
function out = smoothTraj(t,curveDataR)

    % Call evalSmoothTrajectory function
    out = evalSmoothTrajectory(curveDataR,t);

end

== matlab function walkingRobotUtils/Evaluate Smooth Trajectory ==
  data: t input; out output; curveData parameter
function out = smoothTraj(t,curveData)

    % Call evalSmoothTrajectory function
    out = evalSmoothTrajectory(curveData,t);

end

== matlab function walkingRobotUtils/Evaluate Smooth TrajectoryL ==
  data: t input; out output; curveDataL parameter
function out = smoothTraj(t,curveDataL)

    % Call evalSmoothTrajectory function
    out = evalSmoothTrajectory(curveDataL,t);

end
